simulink model "xiti4_8_10T2"  (Simulink 5.0)
settings: Solver=ode45  StartTime=0.0  StopTime=50  FixedStep=0.01  RelTol=1e-3
libraries: simulink_extras x2
CloseFcn:
  | rtwprivate ssgensfun ModelCloseRequest PID_PI
settings Model: LastModifiedBy=ThinkPad

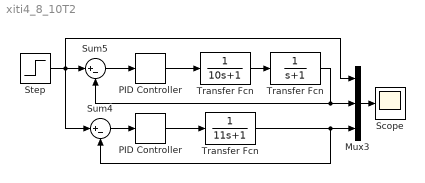
== system xiti4_8_10T2 ==
  " Transfer Fcn" : TransferFcn  Denominator=[1 1]
  Mux3 : Mux  Inputs=3
  PID Controller : simulink_extras/Additional Linear/PID Controller  P=1  I=0  D=0
  "PID Controller " : simulink_extras/Additional Linear/PID Controller  P=1  I=0  D=0
  "Scope " : Scope
      settings: TimeRange=20.2729044834308  YMin=0.36128  YMax=0.809451  SaveName=xiti4_82  DataFormat=Array  MaxDataPoints=500000
  Step : Step  Time=0  SampleTime=0
  Sum4 : Sum  Inputs=|+-  SaturateOnIntegerOverflow=on
  Sum5 : Sum  Inputs=|+-  SaturateOnIntegerOverflow=on
  Transfer Fcn : TransferFcn  Denominator=[10 1]
  "Transfer Fcn " : TransferFcn  Denominator=[11 1]
  wires:
  Step/1 -> Sum5/1, Sum4/1, Mux3/1
  Sum5/1 -> "PID Controller "/1
  "PID Controller "/1 -> Transfer Fcn/1
  Transfer Fcn/1 -> " Transfer Fcn"/1
  Sum4/1 -> PID Controller/1
  PID Controller/1 -> "Transfer Fcn "/1
  Mux3/1 -> "Scope "/1
  " Transfer Fcn"/1 -> Sum5/2, Mux3/2
  "Transfer Fcn "/1 -> Sum4/2, Mux3/3
